simulink model "moonlander_man"  (R2025a)
settings: Solver=ode2  StartTime=0.0  StopTime=Tf  FixedStep=0.1  RelTol=1e-3
values from neighbouring files (symbols this model uses):
  gamma = 6.6743e-11    [pramaters.m]    (also in rl_init_parameters.m)
  h0 = 10e3    (= 10000)    [pramaters.m]    (also in rl_init_parameters.m)
  K = place(A,B,poles)    [pramaters.m]    (also in rl_init_parameters.m)
  M = 7.346e22    (= 7.346e+22)    [pramaters.m]    (also in rl_init_parameters.m)
  m0 = m0_sol + m0_fuel    (= 10000)    [pramaters.m]    (also in rl_init_parameters.m)
  m0_fuel = 8e3    (= 8000)    [pramaters.m]    (also in rl_init_parameters.m)
  mdmax = Pmax/2500    (= 18)    [pramaters.m]    (also in rl_init_parameters.m)
  P_eq_0 = Ff/Pmax*100    (= 36.1114142282)    [pramaters.m]    (also in rl_init_parameters.m)
  Pmax = 45e3    (= 45000)    [pramaters.m]    (also in rl_init_parameters.m)
  R = 3474e3/2    (= 1737000)    [pramaters.m]    (also in rl_init_parameters.m)
  V = inv(C*inv(B*K-A)*B)    [pramaters.m]    (also in rl_init_parameters.m)
undefined symbols (not defined in the file or in its folder): DiscIntNeverNeededParam
libraries: simulink x9, rllib x1
settings Model: PacingRate=3  Creator=grote_w  LastModifiedBy=marcel
settings DataIOCC: SaveOutput=off
settings RTWCC: BuildConfiguration=Faster Runs  GPUComputeCapability=3.5

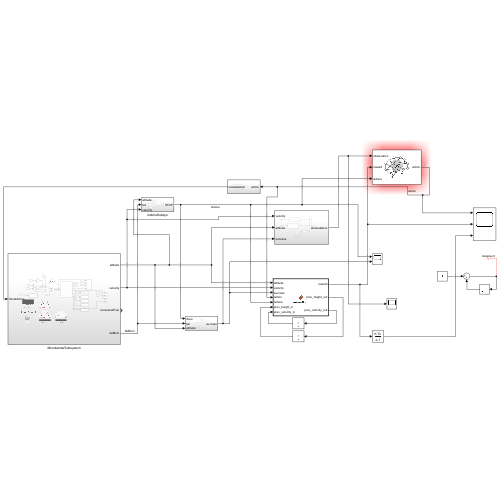
[thumbnail: Simulink's stored preview of the top-level diagram]
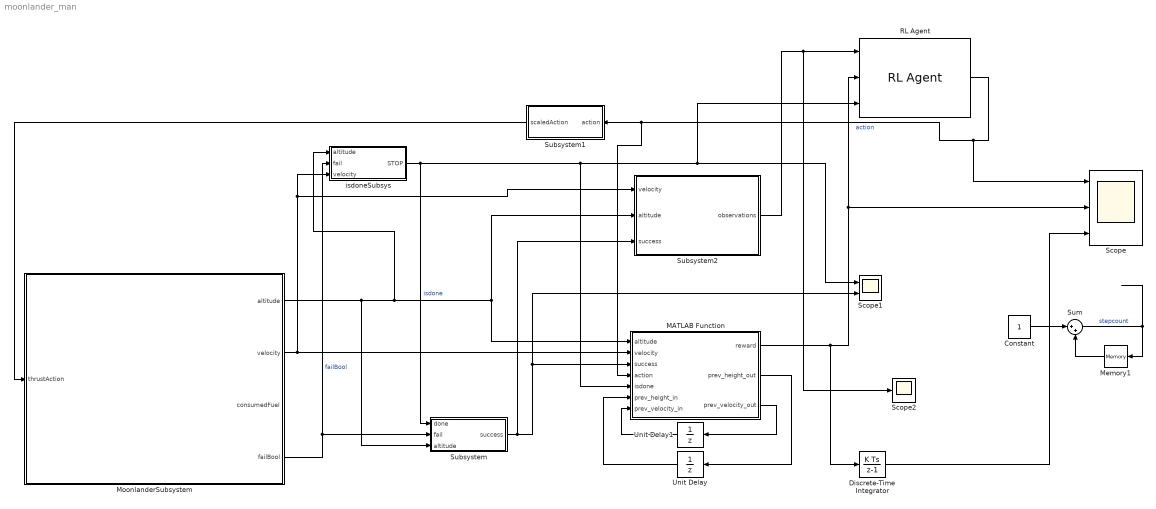
== system moonlander_man ==
  Constant : Constant
  Discrete-Time Integrator : DiscreteIntegrator  SampleTime=-1  ICPrevOutput=DiscIntNeverNeededParam  ICPrevScaledInput=DiscIntNeverNeededParam
  MATLAB Function : MATLAB Function  TreatAsAtomicUnit=on
  Memory1 : Memory
  MoonlanderSubsystem : Subsystem
  RL Agent : rllib/RL Agent  Agent=agent  ExternalActionAsInput=off  ProvideLastAction=off  ProvideCumRwd=off  TreatAsDirectFeedthrough=on  UseStrictObservationDataTypes=off
  Scope : Scope  NumInputPorts=3
      settings: ActiveDisplayYMinimum=-1.2345805019140244  ActiveDisplayYMaximum=1.217665895819664
  Scope1 : Scope  NumInputPorts=2
      settings: ActiveDisplayYMinimum=-1  ActiveDisplayYMaximum=1  DataLoggingVariableName=ScopeData2
  Scope2 : Scope
      settings: ActiveDisplayYMinimum=-1.1660135387910342  ActiveDisplayYMaximum=0.49992743023604069  DataLoggingVariableName=ScopeData3
  Subsystem : Subsystem
  Subsystem1 : Subsystem
  Subsystem2 : Subsystem
  Sum : Sum  Inputs=|++
  Unit Delay : UnitDelay  SampleTime=-1  HasFrameUpgradeWarning=on
  Unit Delay1 : UnitDelay  SampleTime=-1  HasFrameUpgradeWarning=on
  isdoneSubsys : Subsystem
  wires:
  isdoneSubsys/1(STOP) -> Subsystem/1(done), MATLAB Function/5(isdone), Scope1/1, RL Agent/3  "isdone"
  MoonlanderSubsystem/4(failBool) -> Subsystem/2(fail), isdoneSubsys/2(fail)  "failBool"
  MoonlanderSubsystem/2(velocity) -> MATLAB Function/2(velocity), Subsystem2/1(velocity), isdoneSubsys/3(velocity)
  MoonlanderSubsystem/1(altitude) -> Subsystem/3(altitude), MATLAB Function/1(altitude), Subsystem2/2(altitude), isdoneSubsys/1(altitude)
  RL Agent/1 -> Scope/1, MATLAB Function/4(action), Subsystem1/1(action)  "action"
  Constant/1 -> Sum/1
  Sum/1 -> Memory1/1  "stepcount"
  Memory1/1 -> Sum/2
  MATLAB Function/2(prev_height_out) -> Unit Delay/1
  Subsystem/1(success) -> Subsystem2/3(success), Scope1/2, MATLAB Function/3(success)
  MATLAB Function/1(reward) -> Discrete-Time Integrator/1, RL Agent/2, Scope/2
  Subsystem2/1(observations) -> Scope2/1, RL Agent/1
  Subsystem1/1(scaledAction) -> MoonlanderSubsystem/1(thrustAction)
  MATLAB Function/3(prev_velocity_out) -> Unit Delay1/1
  Unit Delay1/1 -> MATLAB Function/7(prev_velocity_in)
  Unit Delay/1 -> MATLAB Function/6(prev_height_in)
  Discrete-Time Integrator/1 -> Scope/3

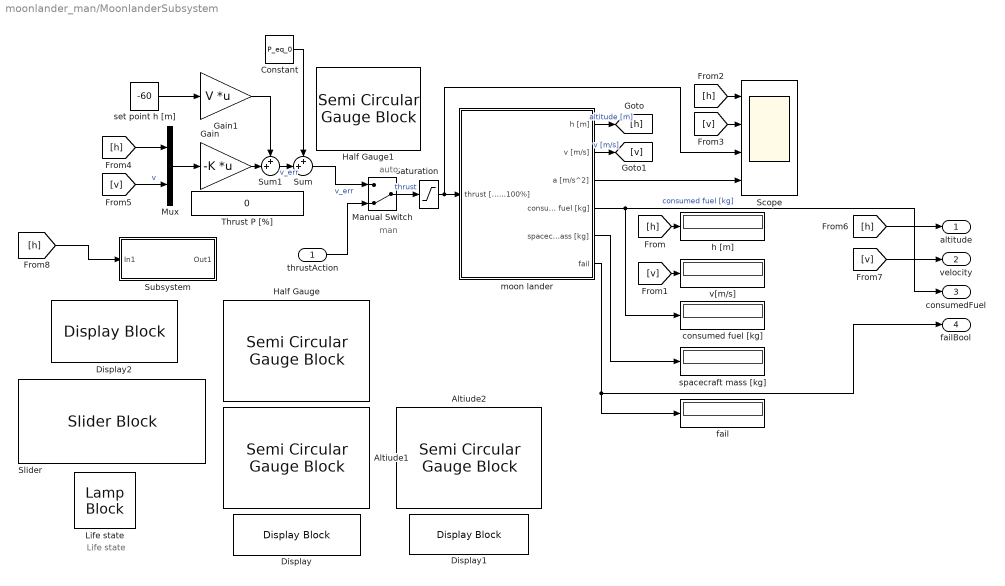
== system moonlander_man/MoonlanderSubsystem ==
  note: Life state
  note: man
  note: auto
  thrustAction : Inport
  Altiude1 : SemiCircularGaugeBlock  ScaleMax=200  FontColor=[0.0, 0.0, 0.0]
  Altiude2 : SemiCircularGaugeBlock  ScaleMin=-120  ScaleMax=20  FontColor=[0.0, 0.0, 0.0]
  Constant : Constant  Value=P_eq_0
  Display : DisplayBlock  LabelPosition=Bottom  Format=Integer  Transparency=1  GridColor=[0.502, 0.502, 0.502]
  Display1 : DisplayBlock  LabelPosition=Bottom  Format=Integer  Transparency=1  GridColor=[0.502, 0.502, 0.502]
  Display2 : DisplayBlock  LabelPosition=Bottom  Format=Integer  Transparency=1  GridColor=[0.502, 0.502, 0.502]
  Gain : Gain  Gain=-K  Multiplication=Matrix(K*u)
  Gain1 : Gain  Gain=V  Multiplication=Matrix(K*u)
  Half Gauge : SemiCircularGaugeBlock  ScaleMax=10  FontColor=[0.0, 0.0, 0.0]
  Half Gauge1 : SemiCircularGaugeBlock  FontColor=[0.0, 0.0, 0.0]
  Life state : LampBlock  LabelPosition=Hide  DefaultColor=[150.0, 150.0, 150.0]
  Manual Switch : ManualSwitch  CurrentSetting=0
  Mux : Mux  Inputs=2
  Saturation : Saturate  UpperLimit=100  LowerLimit=0
  Scope : Scope  NumInputPorts=4
      settings: TimeSpan=80  Title=altitude  ActiveDisplayYMinimum=-1249.97985691733  ActiveDisplayYMaximum=11249.997761879704  YLabel=m
  Slider : SliderBlock
  Subsystem : Subsystem
  Sum : Sum  Inputs=++|
  Sum1 : Sum  Inputs=++|
  Thrust P [%] : Constant  Value=0
  consumed fuel [kg] : Display
  fail : Display
  h [m] : Display
  moon lander : Subsystem
  set point h [m] : Constant  Value=-60
  spacecraft mass [kg] : Display
  v[m/s] : Display
  altitude : Outport
  velocity : Outport  Port=2
  consumedFuel : Outport  Port=3
  failBool : Outport  Port=4
  wires:
  Constant/1 -> Sum/1
  [v] -> Scope/2
  Sum/1 -> Manual Switch/1  "v_err"
  moon lander/6(fail) -> fail/1, failBool/1
  Sum1/1 -> Sum/2  "v_err"
  set point h [m]/1 -> Gain1/1
  moon lander/3(a [m/s^2]) -> Scope/4
  Gain/1 -> Sum1/2
  [h] -> h [m]/1
  [h] -> Mux/1
  moon lander/1(h [m]) -> [h]  "altitude [m]"
  moon lander/5(spacecraft total mass [kg]) -> spacecraft mass [kg]/1
  Saturation/1 -> moon lander/1(thrust [0...100%]), Scope/3
  [h] -> Scope/1
  moon lander/4(consumed fuel [kg]) -> consumedFuel/1, consumed fuel [kg]/1  "consumed fuel [kg]"
  Mux/1 -> Gain/1
  Gain1/1 -> Sum1/1
  moon lander/2(v [m/s]) -> [v]  "v [m/s]"
  Manual Switch/1 -> Saturation/1  "thrust"
  [v] -> Mux/2  "v"
  [v] -> v[m/s]/1
  [h] -> altitude/1
  [v] -> velocity/1
  [h] -> Subsystem/1(In1)
  thrustAction/1 -> Manual Switch/2

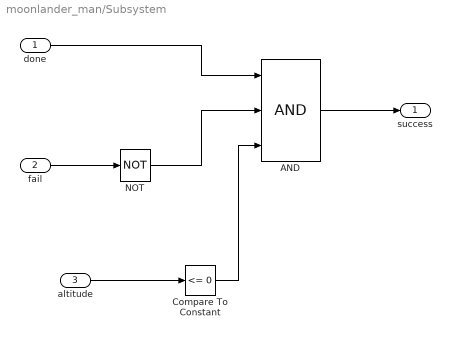
== system moonlander_man/Subsystem ==
  done : Inport
  fail : Inport  Port=2
  altitude : Inport  Port=3
  AND : Logic  Inputs=3  IconShape=distinctive  AllPortsSameDT=off  OutDataTypeStr=boolean
  Compare To Constant : simulink/Logic and Bit Operations/Compare To Constant  relop=<=  const=0  OutDataTypeStr=boolean
  NOT : Logic  Operator=NOT  IconShape=distinctive  AllPortsSameDT=off  OutDataTypeStr=boolean
  success : Outport
  wires:
  AND/1 -> success/1
  done/1 -> AND/1
  fail/1 -> NOT/1
  NOT/1 -> AND/2
  altitude/1 -> Compare To Constant/1
  Compare To Constant/1 -> AND/3

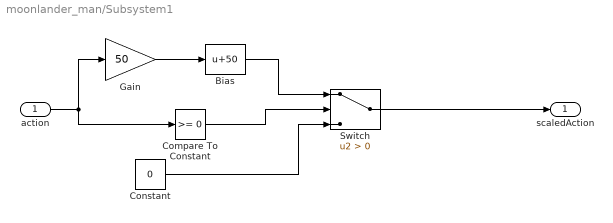
== system moonlander_man/Subsystem1 ==
  action : Inport
  Bias : Bias  Bias=50  SaturateOnIntegerOverflow=off
  Compare To Constant : simulink/Logic and Bit Operations/Compare To Constant  relop=>=  const=0  OutDataTypeStr=boolean
  Constant : Constant  Value=0
  Gain : Gain  Gain=50
  Switch : Switch  Criteria=u2 > Threshold  SaturateOnIntegerOverflow=off  InputSameDT=off
  scaledAction : Outport
  wires:
  Compare To Constant/1 -> Switch/2
  action/1 -> Gain/1, Compare To Constant/1
  Gain/1 -> Bias/1
  Constant/1 -> Switch/3
  Switch/1 -> scaledAction/1
  Bias/1 -> Switch/1

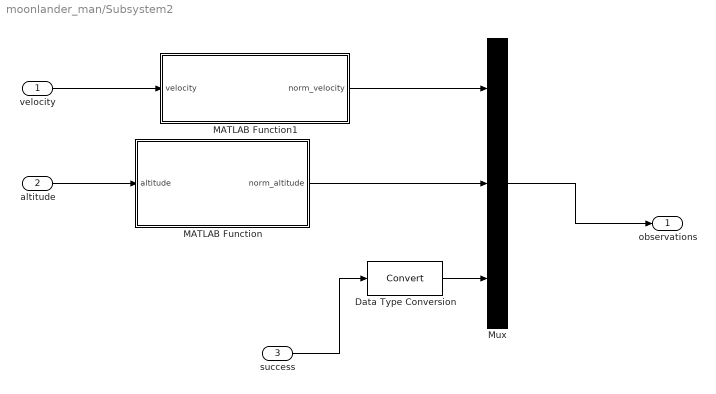
== system moonlander_man/Subsystem2 ==
  velocity : Inport
  altitude : Inport  Port=2
  success : Inport  Port=3
  Data Type Conversion : DataTypeConversion  SaturateOnIntegerOverflow=off  RndMeth=Floor
  MATLAB Function : MATLAB Function  TreatAsAtomicUnit=on
  MATLAB Function1 : MATLAB Function  TreatAsAtomicUnit=on
  Mux : Mux  Inputs=3
  observations : Outport
  wires:
  velocity/1 -> MATLAB Function1/1(velocity)
  altitude/1 -> MATLAB Function/1(altitude)
  success/1 -> Data Type Conversion/1
  Mux/1 -> observations/1
  Data Type Conversion/1 -> Mux/3
  MATLAB Function/1(norm_altitude) -> Mux/2
  MATLAB Function1/1(norm_velocity) -> Mux/1

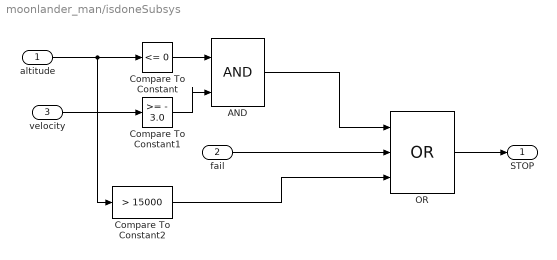
== system moonlander_man/isdoneSubsys ==
  altitude : Inport
  fail : Inport  Port=2
  velocity : Inport  Port=3
  AND : Logic  IconShape=distinctive  AllPortsSameDT=off  OutDataTypeStr=boolean
  Compare To Constant : simulink/Logic and Bit Operations/Compare To Constant  relop=<=  const=0  OutDataTypeStr=boolean
  Compare To Constant1 : simulink/Logic and Bit Operations/Compare To Constant  relop=>=  const=- 3.0  OutDataTypeStr=boolean
  Compare To Constant2 : simulink/Logic and Bit Operations/Compare To Constant  relop=>  const=15000  OutDataTypeStr=boolean
  OR : Logic  Operator=OR  Inputs=3  IconShape=distinctive  AllPortsSameDT=off  OutDataTypeStr=boolean
  STOP : Outport
  wires:
  altitude/1 -> Compare To Constant2/1, Compare To Constant/1
  fail/1 -> OR/2
  velocity/1 -> Compare To Constant1/1
  Compare To Constant1/1 -> AND/2
  Compare To Constant/1 -> AND/1
  AND/1 -> OR/1
  OR/1 -> STOP/1
  Compare To Constant2/1 -> OR/3

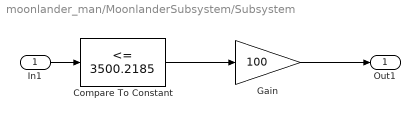
== system moonlander_man/MoonlanderSubsystem/Subsystem ==
  In1 : Inport
  Compare To Constant : simulink/Logic and Bit Operations/Compare To Constant  relop=<=  const=3500.2185  OutDataTypeStr=boolean
  Gain : Gain  Gain=100
  Out1 : Outport
  wires:
  In1/1 -> Compare To Constant/1
  Compare To Constant/1 -> Gain/1
  Gain/1 -> Out1/1

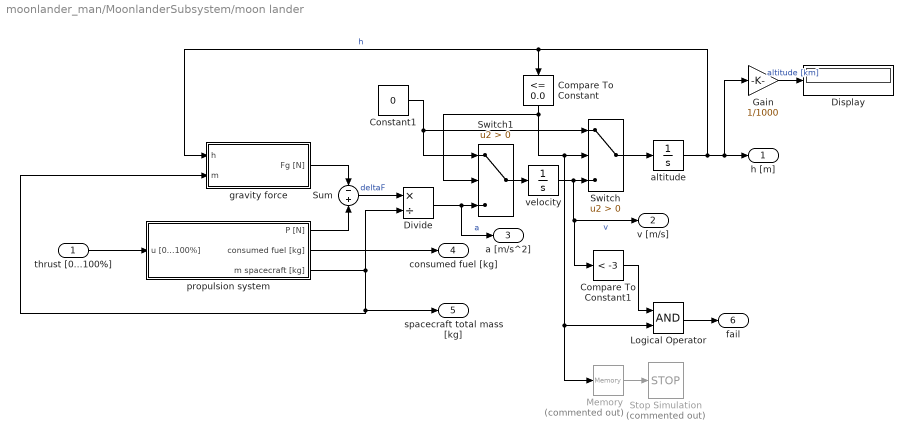
== system moonlander_man/MoonlanderSubsystem/moon lander ==
  thrust [0...100%] : Inport
  Compare To Constant : simulink/Logic and Bit Operations/Compare To Constant  relop=<=  const=0.0  OutDataTypeStr=boolean
  Compare To Constant1 : simulink/Logic and Bit Operations/Compare To Constant  relop=<  const=-3  OutDataTypeStr=boolean
  Constant1 : Constant  Value=0
  Display : Display
  Divide : Product  Inputs=*/
  Gain : Gain  Gain=1/1000
  Logical Operator : Logic  AllPortsSameDT=off  OutDataTypeStr=boolean
  Memory : Memory  Commented=on
  Stop Simulation : Stop  Commented=on
  Sum : Sum  Inputs=-+
  Switch : Switch  Criteria=u2 > Threshold  SaturateOnIntegerOverflow=off  InputSameDT=off
  Switch1 : Switch  Criteria=u2 > Threshold  SaturateOnIntegerOverflow=off  InputSameDT=off
  altitude : Integrator  InitialCondition=h0
  gravity force : Subsystem
  propulsion system : Subsystem
  velocity : Integrator
  h [m] : Outport
  v [m/s] : Outport  Port=2
  a [m/s^2] : Outport  Port=3
  consumed fuel [kg] : Outport  Port=4
  spacecraft total mass [kg] : Outport  Port=5
  fail : Outport  Port=6
  wires:
  Constant1/1 -> Switch/1, Switch1/1
  velocity/1 -> Compare To Constant1/1, v [m/s]/1, Switch/3  "v"
  Compare To Constant/1 -> Switch1/2, Memory/1, Logical Operator/2, Switch/2
  Sum/1 -> Divide/1  "deltaF"
  altitude/1 -> Gain/1, h [m]/1, Compare To Constant/1, gravity force/1(h)  "h"
  gravity force/1(Fg [N]) -> Sum/1
  propulsion system/3(m spacecraft [kg]) -> gravity force/2(m), spacecraft total mass [kg]/1, Divide/2
  Switch/1 -> altitude/1
  Switch1/1 -> velocity/1
  propulsion system/2(consumed fuel [kg]) -> consumed fuel [kg]/1
  propulsion system/1(P [N]) -> Sum/2
  Divide/1 -> a [m/s^2]/1, Switch1/3  "a"
  thrust [0...100%]/1 -> propulsion system/1(u [0...100%])
  Compare To Constant1/1 -> Logical Operator/1
  Logical Operator/1 -> fail/1
  Memory/1 -> Stop Simulation/1
  Gain/1 -> Display/1  "altitude [km]"

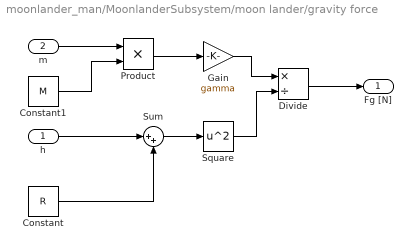
== system moonlander_man/MoonlanderSubsystem/moon lander/gravity force ==
  h : Inport
  m : Inport  Port=2
  Constant : Constant  Value=R
  Constant1 : Constant  Value=M
  Divide : Product  Inputs=*/
  Gain : Gain  Gain=gamma
  Product : Product
  Square : Math  Operator=square
  Sum : Sum  Inputs=|++
  Fg [N] : Outport
  wires:
  h/1 -> Sum/1
  Constant/1 -> Sum/2
  Constant1/1 -> Product/2
  m/1 -> Product/1
  Product/1 -> Gain/1
  Sum/1 -> Square/1
  Gain/1 -> Divide/1
  Square/1 -> Divide/2
  Divide/1 -> Fg [N]/1

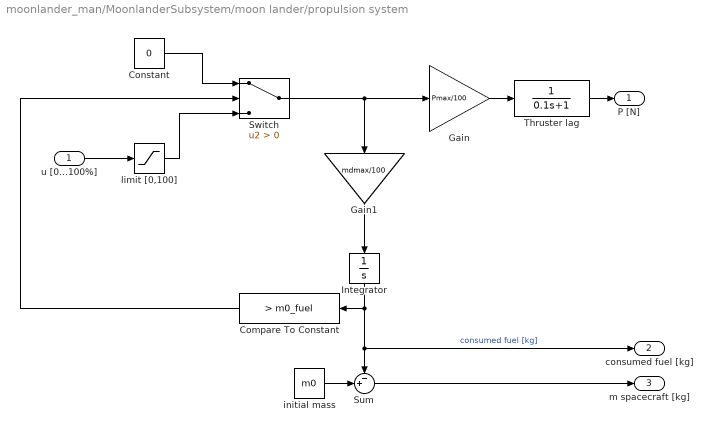
== system moonlander_man/MoonlanderSubsystem/moon lander/propulsion system ==
  u [0...100%] : Inport
  Compare To Constant : simulink/Logic and Bit Operations/Compare To Constant  relop=>  const=m0_fuel  OutDataTypeStr=boolean
  Constant : Constant  Value=0
  Gain : Gain  Gain=Pmax/100
  Gain1 : Gain  Gain=mdmax/100
  Integrator : Integrator  UpperSaturationLimit=m0_fuel  LowerSaturationLimit=0
  Sum : Sum  Inputs=-+|
  Switch : Switch  Criteria=u2 > Threshold  SaturateOnIntegerOverflow=off  InputSameDT=off
  Thruster lag : TransferFcn  Denominator=[0.1 1]
  initial mass : Constant  Value=m0
  limit [0,100] : Saturate  UpperLimit=100  LowerLimit=0
  P [N] : Outport
  consumed fuel [kg] : Outport  Port=2
  m spacecraft [kg] : Outport  Port=3
  wires:
  Gain/1 -> Thruster lag/1
  Switch/1 -> Gain/1, Gain1/1
  Thruster lag/1 -> P [N]/1
  initial mass/1 -> Sum/2
  Sum/1 -> m spacecraft [kg]/1
  Integrator/1 -> Compare To Constant/1, consumed fuel [kg]/1, Sum/1  "consumed fuel [kg]"
  Gain1/1 -> Integrator/1
  Compare To Constant/1 -> Switch/2
  u [0...100%]/1 -> limit [0,100]/1
  Constant/1 -> Switch/1
  limit [0,100]/1 -> Switch/3

== matlab function moonlander_man/Subsystem2/MATLAB Function ==
  data: altitude input; norm_altitude output
function norm_altitude = fcn(altitude)
    
    max_altitude = 15000;
    min_altitude = 0;
    
    % normalize alt & vel [-1, 1]
    norm_altitude = 2 * ((altitude - min_altitude) / (max_altitude - min_altitude)) - 1;

end

== matlab function moonlander_man/MATLAB Function ==
  data: altitude input; reward output; velocity input; success input; action input; isdone input; prev_height_in input; prev_velocity_in input; prev_height_out output; prev_velocity_out output
function [reward, prev_height_out, prev_velocity_out]= rewardFcn(altitude, velocity, success, action, isdone, prev_height_in, prev_velocity_in)
    
    %max_altitude = 15000;
    %min_altitude = 0;
    %max_abs_velocity = 180;
    %min_abs_velocity = -180;
    threshold_height = 3500.2185;
    reward = 0;
    
    % action reward
    if altitude <= threshold_height
        if action > 0
            reward = reward + 1;
        else 
            reward = reward -1;
        end
    else
        if action <= 0
            reward = reward +1;
        else
            reward = reward -1;
        end
    end
    
    % height error reward
    if prev_height_in > altitude
        reward = reward +1;
    else
        reward = reward -1;
    end

    %velocity reward
    if altitude > threshold_height
        if velocity < prev_velocity_in
            reward = reward + 1;
        else
            reward = reward -1;
        end
    else 
        if (velocity > prev_velocity_in) && (velocity <= 0)
            reward = reward + 1;
        else
            reward = reward - 1;
        end
    end

    %ascending penalty
    if (altitude <= threshold_height) && (altitude >= 3)
        if altitude > prev_height_in
            reward = -3;
        end
    end

    %final reward
    if isdone
        if success
            reward = reward + 10000;
        else
            reward = reward - 1000;
        end 
    end

    prev_height_out = altitude;
    prev_velocity_out = velocity;
   
end

== matlab function moonlander_man/Subsystem2/MATLAB Function1 ==
  data: velocity input; norm_velocity output
function norm_velocity = fcn(velocity)

    max_abs_velocity = 180;
    min_abs_velocity = -180;
    
    % normalize alt & vel [-1, 1]
    norm_velocity = 2 * ((velocity - min_abs_velocity) / (max_abs_velocity - min_abs_velocity)) -1;

end
